simulink model "FLIGHT_Hexacopter_fail"  (R2024a)
settings: Solver=FixedStepDiscrete  StartTime=0.0  StopTime=inf  FixedStep=SampleTime  RelTol=1e-3  EnableMultiTasking=on
InitFcn:
  | Init_FLIGHT_Hexacopter
values from neighbouring files (symbols this model uses):
  Kdpr = 0.004    [Init_FLIGHT_Hexacopter_fromNCMS.m]
  Kdrr = 0.004    [Init_FLIGHT_Hexacopter_fromNCMS.m]
  Kdvz = 0.0254    [Init_FLIGHT_Hexacopter_fromNCMS.m]
  Kdyr = 0.0298    [Init_FLIGHT_Hexacopter_fromNCMS.m]
  Kipr = 0.0    (= 0)    [Init_FLIGHT_Hexacopter_fromNCMS.m]
  Kirr = 0.0    (= 0)    [Init_FLIGHT_Hexacopter_fromNCMS.m]
  Kivz = 0.6304    [Init_FLIGHT_Hexacopter_fromNCMS.m]
  Kiyr = 0.0    (= 0)    [Init_FLIGHT_Hexacopter_fromNCMS.m]
  Kpp = 3.3894    [Init_FLIGHT_Hexacopter_fromNCMS.m]
  Kppr = 0.1    [Init_FLIGHT_Hexacopter_fromNCMS.m]
  Kpr = 3.3894    [Init_FLIGHT_Hexacopter_fromNCMS.m]
  Kprr = 0.1    [Init_FLIGHT_Hexacopter_fromNCMS.m]
  Kpvz = 0.3191    [Init_FLIGHT_Hexacopter_fromNCMS.m]
  Kpyr = 0.3744    [Init_FLIGHT_Hexacopter_fromNCMS.m]
  MAX_CONTROL_ANGLE_PITCH = 30*pi/180    (= 0.523598775598)    [Init_FLIGHT_Hexacopter.m]    (also in Init_FLIGHT_Hexacopter_fromNCMS.m = 0.349065850399)
  MAX_CONTROL_ANGLE_RATE_PITCH = 360*pi/180    (= 6.28318530718)    [Init_FLIGHT_Hexacopter.m]    (also in Init_FLIGHT_Hexacopter_fromNCMS.m)
  MAX_CONTROL_ANGLE_RATE_ROLL = 360*pi/180    (= 6.28318530718)    [Init_FLIGHT_Hexacopter.m]    (also in Init_FLIGHT_Hexacopter_fromNCMS.m)
  MAX_CONTROL_ANGLE_RATE_Y = 120*pi/180    (= 2.09439510239)    [Init_FLIGHT_Hexacopter.m]    (also in Init_FLIGHT_Hexacopter_fromNCMS.m)
  MAX_CONTROL_ANGLE_ROLL = 30*pi/180    (= 0.523598775598)    [Init_FLIGHT_Hexacopter.m]    (also in Init_FLIGHT_Hexacopter_fromNCMS.m = 0.349065850399)
  MAX_CONTROL_VELOCITY_Z = 1    [Init_FLIGHT_Hexacopter.m]    (also in Init_FLIGHT_Hexacopter_fromNCMS.m)
  Npr = 50    [Init_FLIGHT_Hexacopter_fromNCMS.m]
  Nrr = 50    [Init_FLIGHT_Hexacopter_fromNCMS.m]
  Nvz = Npr    (= 50)    [Init_FLIGHT_Hexacopter_fromNCMS.m]
  Nyr = 50    [Init_FLIGHT_Hexacopter_fromNCMS.m]
  SampleTime = 1/250    (= 0.004)    [Init_FLIGHT_Hexacopter.m]    (also in Init_FLIGHT_Hexacopter_fromNCMS.m = 0.01)
  THR_HOVER = 0.6085    [Init_FLIGHT_Hexacopter_fromNCMS.m]
libraries: px4lib x7, slpidlib x6, px4Sensorslib x3, simulink x2, px4uORBlib x1
(part 1 of 2)
settings Model: ExtModeTrigDuration=10  Creator=user  LastModifiedBy=user
settings SolverCC: PositivePriorityOrder=on
settings OptimizationCC: DefaultUnderspecifiedDataType=single  EnhancedBackFolding=on  PassReuseOutputArgsAs=Individual arguments  ZeroExternalMemoryAtStartup=off  ZeroInternalMemoryAtStartup=off  MaxStackSize=64  OptimizeBlockOrder=speed  DifferentSizesBufferReuse=on  OptimizationCustomize=off  EfficientTunableParamExpr=on
settings DebuggingCC: ParameterTunabilityLossMsg=error  UnconnectedInputMsg=warning  UnconnectedOutputMsg=warning  UnconnectedLineMsg=warning
settings HardwareCC: ProdBitPerPointer=32  ProdBitPerSizeT=32  ProdBitPerPtrDiffT=32  ProdLargestAtomicInteger=Long  ProdLargestAtomicFloat=Double  ProdWordSize=32  ProdLongLongMode=on  ProdHWDeviceType=ARM Compatible->ARM Cortex
settings ModelReferenceCC: EnableRefExpFcnMdlSchedulingChecks=on
settings SFSimCC: MATLABDynamicMemAlloc=off  SimTargetLang=C++
settings RTWCC: Description=Embedded Coder  SystemTargetFile=ert.tlc  HardwareBoard=PX4 Cube Orange  TLCOptions="-aInlineSetEventsForThisBaseRateFcn=TLC_FALSE -aSuppressMultiTaskScheduler=TLC_FALSE  -aRateBasedStepFcn=0"  TemplateMakefile=ert_default_tmf  Toolchain=GNU Tools for PX4 Autopilots  TargetLang=C++  GPUComputeCapability=3.5  DLArmComputeVersion=19.05
settings CodeAppCC: ForceParamTrailComments=on  IgnoreCustomStorageClasses=off  OperatorAnnotations=on  SimulinkDataObjDesc=on  SFDataObjDesc=on  InsertBlockDesc=on
settings ERTTargetCC: MatFileLogging=on  ExtModeTransport=3  ExtModeStaticAlloc=on  ExtModeStaticAllocSize=1024  ExtModeMexFile=ext_xcp  ExtModeIntrfLevel=Level2 - Open

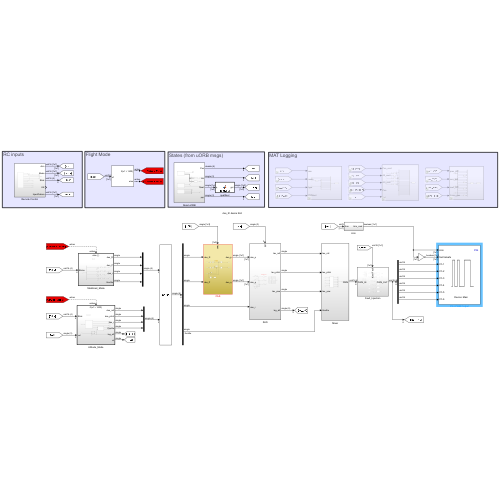
[thumbnail: Simulink's stored preview of the top-level diagram]
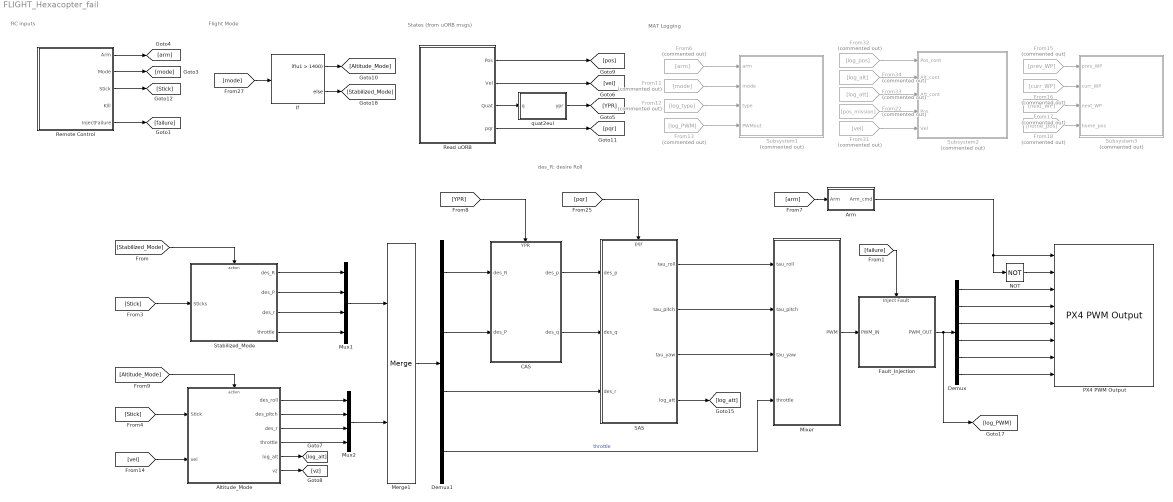
== system FLIGHT_Hexacopter_fail ==
  note: des_R: desire Roll
  note: MAT Logging
  note: States (from uORB msgs)
  note: RC inputs
  note: Flight Mode
  Altitude_Mode : Subsystem
  Arm : Subsystem
  CAS : Subsystem
      settings: PortSchema="{\"entries\":[{\"content\":{\"sides\":[{\"content\":{\"connectorIds\":[\"In1\",\"In2\"]},\"type\":\"ConnectorPlacement.EquallySpacedRectSide\",\"uuid\":\"cd8887f4-d1ed-4900-9f4b-1d4d1f8b3f25\"},{\"content\":{\"connectorIds\":[\"Out1\",\"Out2\"],\"side\":\"RIGHT\"},\"type\":\"ConnectorPlacement.EquallySpacedRectSide\",\"uuid\":\"04130072-6486-422d-805d-1cc854b52651\"},{\"content\":{\"connectorIds\":[\"In3\"],\"side\":\"TOP\"},\"type\":\"ConnectorPlacement.EquallySpacedRectSide\",\"uuid\":\"bd75db6e-c74e-4c5f-b850-7d60a52ba57c\"}]},\"type\":\"ConnectorPlacement.EquallySpacedConnector\",\"uuid\":\"0b75b304-9bf2-4ad4-968c-84bda26ed250\"}],\"packageUris\":[\"http://schema.mathworks.com/mf0/Connector/R2020b\"],\"version\":\"1.0\"}"
  Demux : Demux  Outputs=6
  Demux1 : Demux
  Fault_Injection : Subsystem
      settings: PortSchema="{\"entries\":[{\"content\":{\"sides\":[{\"content\":{\"connectorIds\":[\"In1\"]},\"type\":\"ConnectorPlacement.EquallySpacedRectSide\",\"uuid\":\"fab26c65-8d77-46b7-b375-2033d08e8306\"},{\"content\":{\"connectorIds\":[\"Out1\"],\"side\":\"RIGHT\"},\"type\":\"ConnectorPlacement.EquallySpacedRectSide\",\"uuid\":\"bc3f50bd-e170-4b75-8089-4f92da68e83e\"},{\"content\":{\"connectorIds\":[\"In2\"],\"side\":\"TOP\"},\"type\":\"ConnectorPlacement.EquallySpacedRectSide\",\"uuid\":\"873ada90-6f93-48ab-a701-a52d28357753\"}]},\"type\":\"ConnectorPlacement.EquallySpacedConnector\",\"uuid\":\"201be8b3-bff4-4924-8e0c-28e5fee33d1c\"}],\"packageUris\":[\"http://schema.mathworks.com/mf0/Connector/R2020b\"],\"version\":\"1.0\"}"
  From11 : From  Commented=on  GotoTag=mode
  From12 : From  Commented=on  GotoTag=log_type
  From13 : From  Commented=on  GotoTag=log_PWM
  From15 : From  Commented=on  GotoTag=prev_WP
  From16 : From  Commented=on  GotoTag=curr_WP
  From17 : From  Commented=on  GotoTag=next_WP
  From18 : From  Commented=on  GotoTag=home_pos
  From22 : From  Commented=on  GotoTag=pos_mission
  From31 : From  Commented=on  GotoTag=vel
  From32 : From  Commented=on  GotoTag=log_pos
  From33 : From  Commented=on  GotoTag=log_att
  From34 : From  Commented=on  GotoTag=log_alt
  From6 : From  Commented=on  GotoTag=arm
  If : If  IfExpression=u1 > 1400
  Merge1 : Merge
  Mixer : Subsystem
  Mux1 : Mux
  Mux2 : Mux
  NOT : Logic  Operator=NOT  IconShape=distinctive  AllPortsSameDT=off  OutDataTypeStr=boolean
  PX4 PWM Output : px4lib/PX4 PWM Output  pwmDevice=Main  pwmChannel1_=on  pwmChannel2_=on  pwmChannel3_=on  pwmChannel4_=on  pwmChannel5_=on  pwmChannel6_=on  pwmChannel7_=off  pwmChannel8_=off
  Read uORB : Subsystem
  Remote Control : Subsystem
  SAS : Subsystem
      settings: PortSchema="{\"entries\":[{\"content\":{\"sides\":[{\"content\":{\"connectorIds\":[\"In1\",\"In2\",\"In3\"]},\"type\":\"ConnectorPlacement.EquallySpacedRectSide\",\"uuid\":\"77bb8164-b871-4593-8031-335c6110c17c\"},{\"content\":{\"connectorIds\":[\"Out1\",\"Out2\",\"Out3\",\"Out4\"],\"side\":\"RIGHT\"},\"type\":\"ConnectorPlacement.EquallySpacedRectSide\",\"uuid\":\"f99d9e85-7cc9-4d0a-ad5d-789571e28028\"},{\"content\":{\"connectorIds\":[\"In4\"],\"side\":\"TOP\"},\"type\":\"ConnectorPlacement.EquallySpacedRectSide\",\"uuid\":\"174eb658-0f52-43c7-ba1a-1a337b4835ca\"}]},\"type\":\"ConnectorPlacement.EquallySpacedConnector\",\"uuid\":\"7932b1f4-42ae-4dcf-8815-0888db42261d\"}],\"packageUris\":[\"http://schema.mathworks.com/mf0/Connector/R2020b\"],\"version\":\"1.0\"}"
  Stabilized_Mode : Subsystem  TreatAsAtomicUnit=on
  Subsystem1 : Subsystem  Commented=on
  Subsystem2 : Subsystem  Commented=on
  Subsystem3 : Subsystem  Commented=on
  quat2eul : MATLAB Function  TreatAsAtomicUnit=on
  wires:
  Demux/1 -> PX4 PWM Output/3
  Demux/2 -> PX4 PWM Output/4
  Demux/3 -> PX4 PWM Output/5
  Demux/4 -> PX4 PWM Output/6
  NOT/1 -> PX4 PWM Output/2
  Read uORB/3(Quat) -> quat2eul/1(q)
  Arm/1(Arm_cmd) -> NOT/1, PX4 PWM Output/1
  Read uORB/2(Vel) -> [vel]
  Remote Control/3(Stick) -> [Stick]
  Remote Control/2(Mode) -> [mode]
  Remote Control/1(Arm) -> [arm]
  Read uORB/1(Pos) -> [pos]
  Merge1/1 -> Demux1/1
  [arm] -> Arm/1(Arm)
  quat2eul/1(ypr) -> [YPR]
  Read uORB/4(pqr) -> [pqr]
  SAS/4(log_att) -> [log_att]
  From6/1 -> Subsystem1/1(arm)
  From11/1 -> Subsystem1/2(mode)
  From12/1 -> Subsystem1/3(type)
  From13/1 -> Subsystem1/4(PWMout)
  [pqr] -> SAS/4(pqr)
  From31/1 -> Subsystem2/5(Vel)
  From22/1 -> Subsystem2/4(Pos)
  From33/1 -> Subsystem2/3(Att_cont)
  From34/1 -> Subsystem2/2(Alt_cont)
  From32/1 -> Subsystem2/1(Pos_cont)
  From18/1 -> Subsystem3/4(home_pos)
  From17/1 -> Subsystem3/3(next_WP)
  From16/1 -> Subsystem3/2(curr_WP)
  From15/1 -> Subsystem3/1(prev_WP)
  Demux/5 -> PX4 PWM Output/7
  Demux/6 -> PX4 PWM Output/8
  [mode] -> If/1
  Demux1/2 -> CAS/2(des_P)
  Demux1/1 -> CAS/1(des_R)
  [YPR] -> CAS/3(YPR)
  [Stabilized_Mode] -> Stabilized_Mode/Action
  [Stick] -> Stabilized_Mode/1(Sticks)
  Mux1/1 -> Merge1/1
  CAS/1(des_p) -> SAS/1(des_p)
  CAS/2(des_q) -> SAS/2(des_q)
  Demux1/3 -> SAS/3(des_r)
  Demux1/4 -> Mixer/4(throttle)  "throttle"
  [Stick] -> Altitude_Mode/1(Stick)
  [Altitude_Mode] -> Altitude_Mode/Action
  Altitude_Mode/1(des_roll) -> Mux2/1
  Altitude_Mode/2(des_pitch) -> Mux2/2
  Altitude_Mode/3(des_r) -> Mux2/3
  Altitude_Mode/4(throttle) -> Mux2/4
  Mux2/1 -> Merge1/2
  Altitude_Mode/5(log_alt) -> [log_alt]
  Altitude_Mode/6(vz) -> [vz]
  [vel] -> Altitude_Mode/2(vel)
  SAS/1(tau_roll) -> Mixer/1(tau_roll)
  SAS/2(tau_pitch) -> Mixer/2(tau_pitch)
  SAS/3(tau_yaw) -> Mixer/3(tau_yaw)
  Mixer/1(PWM) -> Fault_Injection/1(PWM_IN)
  Fault_Injection/1(PWM_OUT) -> [log_PWM], Demux/1
  Remote Control/5(InjectFailure) -> [failure]
  [failure] -> Fault_Injection/2(Inject Fault)
  If/1 -> [Altitude_Mode]
  If/2 -> [Stabilized_Mode]
  Stabilized_Mode/1(des_R) -> Mux1/1
  Stabilized_Mode/2(des_P) -> Mux1/2
  Stabilized_Mode/3(des_r) -> Mux1/3
  Stabilized_Mode/4(throttle) -> Mux1/4

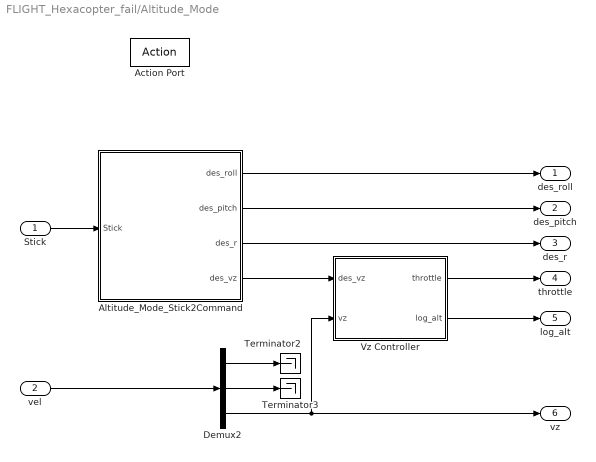
== system FLIGHT_Hexacopter_fail/Altitude_Mode ==
  Stick : Inport
  vel : Inport  Port=2
  Action Port : ActionPort  ActionPortLabel=if(u1 > 1400)
  Altitude_Mode_Stick2Command : Subsystem
  Demux2 : Demux  Outputs=3
  Terminator2 : Terminator
  Terminator3 : Terminator
  Vz Controller : Subsystem
  des_roll : Outport
  des_pitch : Outport  Port=2
  des_r : Outport  Port=3
  throttle : Outport  Port=4
  log_alt : Outport  Port=5
  vz : Outport  Port=6
  wires:
  Stick/1 -> Altitude_Mode_Stick2Command/1(Stick)
  Vz Controller/1(throttle) -> throttle/1
  Demux2/3 -> vz/1, Vz Controller/2(vz)
  Altitude_Mode_Stick2Command/1(des_roll) -> des_roll/1
  vel/1 -> Demux2/1
  Altitude_Mode_Stick2Command/3(des_r) -> des_r/1
  Demux2/1 -> Terminator2/1
  Vz Controller/2(log_alt) -> log_alt/1
  Demux2/2 -> Terminator3/1
  Altitude_Mode_Stick2Command/2(des_pitch) -> des_pitch/1
  Altitude_Mode_Stick2Command/4(des_vz) -> Vz Controller/1(des_vz)

== system FLIGHT_Hexacopter_fail/Arm ==
  Arm : Inport
  Compare To Constant3 : simulink/Logic and Bit Operations/Compare To Constant  relop=>=  const=uint16(1800)  OutDataTypeStr=boolean
  Arm_cmd : Outport  VectorParamsAs1DForOutWhenUnconnected=off
  wires:
  Arm/1 -> Compare To Constant3/1
  Compare To Constant3/1 -> Arm_cmd/1

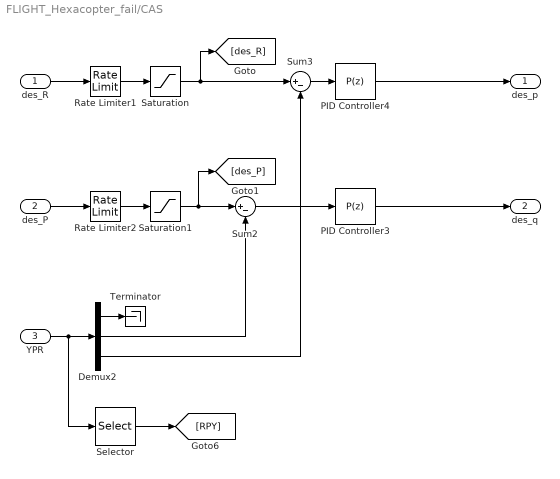
== system FLIGHT_Hexacopter_fail/CAS ==
  des_R : Inport
  des_P : Inport  Port=2
  YPR : Inport  Port=3
  Demux2 : Demux  Outputs=3
  PID Controller3 : slpidlib/PID Controller  Controller=P  Form=Parallel  TimeDomain=Discrete-time  UseExternalTs=off  SampleTime=SampleTime  IntegratorMethod=Forward Euler  FilterMethod=Forward Euler  ControllerParametersSource=internal  P=Kpp  I=1  UseKiTs=off  D=0  UseExternalDerivativeSource=off  N=100  UseFilter=on  TunerSelectOption=Transfer Function Based (PID Tuner App)  InitialConditionSource=internal  InitialConditionForIntegrator=0  InitialConditionForFilter=0  DifferentiatorICPrevScaledInput=0  ExternalReset=none  TrackingMode=off  Kt=1  LimitOutput=on  SatLimitsSource=internal  UpperSaturationLimit=MAX_CONTROL_ANGLE_RATE_PITCH  LowerSaturationLimit=-MAX_CONTROL_ANGLE_RATE_PITCH  LinearizeAsGain=on  AntiWindupMode=none  Kb=1  LimitIntegrator=off  UpperIntegratorSaturationLimit=inf  LowerIntegratorSaturationLimit=-inf  POutMin=[]  POutMax=[]  IOutMin=[]  IOutMax=[]  DOutMin=[]  DOutMax=[]  NOutMin=[]  NOutMax=[]  SumOutMin=[]  SumOutMax=[]  SaturationOutMin=[]  SaturationOutMax=[]  PParamMin=[]  PParamMax=[]  IParamMin=[]  IParamMax=[]  DParamMin=[]  DParamMax=[]  NParamMin=[]  NParamMax=[]  KbParamMin=[]  KbParamMax=[]  KtParamMin=[]  KtParamMax=[]  KbOutMin=[]  KbOutMax=[]  KtOutMin=[]  KtOutMax=[]  IntegratorOutMin=[]  IntegratorOutMax=[]  FilterOutMin=[]  FilterOutMax=[]  SumI1OutMin=[]  SumI1OutMax=[]  SumI2OutMin=[]  SumI2OutMax=[]  SumI3OutMin=[]  SumI3OutMax=[]  SumI4OutMin=[]  SumI4OutMax=[]  SumDOutMin=[]  SumDOutMax=[]  DifferentiatorOutMin=[]  DifferentiatorOutMax=[]  FilterDiffOutCoefMin=[]  FilterDiffOutCoefMax=[]  ReciprocalOutMin=[]  ReciprocalOutMax=[]  SumDenOutMin=[]  SumDenOutMax=[]  SumNumOutMin=[]  SumNumOutMax=[]  DivideOutMin=[]  DivideOutMax=[]  UdiffTsProdOutMin=[]  UdiffTsProdOutMax=[]  NTsProdOutMin=[]  NTsProdOutMax=[]  UintegralTsProdOutMin=[]  UintegralTsProdOutMax=[]  UngainTsProdOutMin=[]  UngainTsProdOutMax=[]  ClampingZeroOutDataTypeStr=Inherit: Inherit via back propagation  ClampingZeroOutMin=[]  ClampingZeroOutMax=[]  FilterDenConstantOutDataTypeStr=Inherit: Inherit via back propagation  FilterDenConstantOutMin=[]  FilterDenConstantOutMax=[]  PCopyOutDataTypeStr=Inherit: Inherit via back propagation  PCopyOutMin=[]  PCopyOutMax=[]  NCopyOutDataTypeStr=Inherit: Inherit via back propagation  NCopyOutMin=[]  NCopyOutMax=[]  IntegratorContinuousStateAttributes=''  IntegratorStateMustResolveToSignalObject=off  IntegratorRTWStateStorageClass=Auto  FilterContinuousStateAttributes=''  FilterStateMustResolveToSignalObject=off  FilterRTWStateStorageClass=Auto  ParallelPVariant=InternalParameters  IdealPVariant=Disabled  IVariant=Disabled  DVariant=Disabled  IntegratorVariant=Disabled  SatVariant=Enabled  AWVariant=Disabled  PCopyVariant=Disabled  TRVariant=Disabled  FdbkBlocksVariant=Forward  IdealPFdbkVariant=Disabled  SatFdbkVariant=Disabled  DerivativeFilterVariant=Disabled  NVariant=Disabled  NCopyVariant=Disabled_SignalSpec  FilterICVariant=Disabled  IntegratorICVariant=Disabled  ExternalResetVariant=Disabled  TRSumVariant=Passthrough  SumFdbkVariant=Disabled  SumVariant=Passthrough_P  TsampFilterVariant=InternalTs  TsampNgainVariant=Passthrough  TsampIntegralVariant=Disabled_SignalSpec  ExternalSaturationOutDataTypeStr=Inherit: Same as second input  DerivativeSourceVariant=Disabled
  PID Controller4 : slpidlib/PID Controller  Controller=P  Form=Parallel  TimeDomain=Discrete-time  UseExternalTs=off  SampleTime=SampleTime  IntegratorMethod=Forward Euler  FilterMethod=Forward Euler  ControllerParametersSource=internal  P=Kpr  I=1  UseKiTs=off  D=0  UseExternalDerivativeSource=off  N=100  UseFilter=on  TunerSelectOption=Transfer Function Based (PID Tuner App)  InitialConditionSource=internal  InitialConditionForIntegrator=0  InitialConditionForFilter=0  DifferentiatorICPrevScaledInput=0  ExternalReset=none  TrackingMode=off  Kt=1  LimitOutput=on  SatLimitsSource=internal  UpperSaturationLimit=MAX_CONTROL_ANGLE_RATE_ROLL  LowerSaturationLimit=-MAX_CONTROL_ANGLE_RATE_ROLL  LinearizeAsGain=on  AntiWindupMode=none  Kb=1  LimitIntegrator=off  UpperIntegratorSaturationLimit=inf  LowerIntegratorSaturationLimit=-inf  POutMin=[]  POutMax=[]  IOutMin=[]  IOutMax=[]  DOutMin=[]  DOutMax=[]  NOutMin=[]  NOutMax=[]  SumOutMin=[]  SumOutMax=[]  SaturationOutMin=[]  SaturationOutMax=[]  PParamMin=[]  PParamMax=[]  IParamMin=[]  IParamMax=[]  DParamMin=[]  DParamMax=[]  NParamMin=[]  NParamMax=[]  KbParamMin=[]  KbParamMax=[]  KtParamMin=[]  KtParamMax=[]  KbOutMin=[]  KbOutMax=[]  KtOutMin=[]  KtOutMax=[]  IntegratorOutMin=[]  IntegratorOutMax=[]  FilterOutMin=[]  FilterOutMax=[]  SumI1OutMin=[]  SumI1OutMax=[]  SumI2OutMin=[]  SumI2OutMax=[]  SumI3OutMin=[]  SumI3OutMax=[]  SumI4OutMin=[]  SumI4OutMax=[]  SumDOutMin=[]  SumDOutMax=[]  DifferentiatorOutMin=[]  DifferentiatorOutMax=[]  FilterDiffOutCoefMin=[]  FilterDiffOutCoefMax=[]  ReciprocalOutMin=[]  ReciprocalOutMax=[]  SumDenOutMin=[]  SumDenOutMax=[]  SumNumOutMin=[]  SumNumOutMax=[]  DivideOutMin=[]  DivideOutMax=[]  UdiffTsProdOutMin=[]  UdiffTsProdOutMax=[]  NTsProdOutMin=[]  NTsProdOutMax=[]  UintegralTsProdOutMin=[]  UintegralTsProdOutMax=[]  UngainTsProdOutMin=[]  UngainTsProdOutMax=[]  ClampingZeroOutDataTypeStr=Inherit: Inherit via back propagation  ClampingZeroOutMin=[]  ClampingZeroOutMax=[]  FilterDenConstantOutDataTypeStr=Inherit: Inherit via back propagation  FilterDenConstantOutMin=[]  FilterDenConstantOutMax=[]  PCopyOutDataTypeStr=Inherit: Inherit via back propagation  PCopyOutMin=[]  PCopyOutMax=[]  NCopyOutDataTypeStr=Inherit: Inherit via back propagation  NCopyOutMin=[]  NCopyOutMax=[]  IntegratorContinuousStateAttributes=''  IntegratorStateMustResolveToSignalObject=off  IntegratorRTWStateStorageClass=Auto  FilterContinuousStateAttributes=''  FilterStateMustResolveToSignalObject=off  FilterRTWStateStorageClass=Auto  ParallelPVariant=InternalParameters  IdealPVariant=Disabled  IVariant=Disabled  DVariant=Disabled  IntegratorVariant=Disabled  SatVariant=Enabled  AWVariant=Disabled  PCopyVariant=Disabled  TRVariant=Disabled  FdbkBlocksVariant=Forward  IdealPFdbkVariant=Disabled  SatFdbkVariant=Disabled  DerivativeFilterVariant=Disabled  NVariant=Disabled  NCopyVariant=Disabled_SignalSpec  FilterICVariant=Disabled  IntegratorICVariant=Disabled  ExternalResetVariant=Disabled  TRSumVariant=Passthrough  SumFdbkVariant=Disabled  SumVariant=Passthrough_P  TsampFilterVariant=InternalTs  TsampNgainVariant=Passthrough  TsampIntegralVariant=Disabled_SignalSpec  ExternalSaturationOutDataTypeStr=Inherit: Same as second input  DerivativeSourceVariant=Disabled
  Rate Limiter1 : RateLimiter  RisingSlewLimit=40*pi/180  FallingSlewLimit=-40*pi/180  SampleTimeMode=inherited
  Rate Limiter2 : RateLimiter  RisingSlewLimit=40*pi/180  FallingSlewLimit=-40*pi/180  SampleTimeMode=inherited
  Saturation : Saturate  UpperLimit=MAX_CONTROL_ANGLE_ROLL  LowerLimit=-MAX_CONTROL_ANGLE_ROLL
  Saturation1 : Saturate  UpperLimit=MAX_CONTROL_ANGLE_PITCH  LowerLimit=-MAX_CONTROL_ANGLE_PITCH
  Selector : Selector  InputPortWidth=3  IndexOptions=Index vector (dialog)  Indices=[3 2 1]  OutputSizes=1
  Sum2 : Sum  Inputs=|+-
  Sum3 : Sum  Inputs=|+-
  Terminator : Terminator
  des_p : Outport
  des_q : Outport  Port=2
  wires:
  des_R/1 -> Rate Limiter1/1
  Saturation/1 -> [des_R], Sum3/1
  Sum3/1 -> PID Controller4/1
  Sum2/1 -> PID Controller3/1
  Saturation1/1 -> [des_P], Sum2/1
  Demux2/3 -> Sum3/2
  Demux2/2 -> Sum2/2
  YPR/1 -> Selector/1, Demux2/1
  Selector/1 -> [RPY]
  Rate Limiter1/1 -> Saturation/1
  Demux2/1 -> Terminator/1
  des_P/1 -> Rate Limiter2/1
  Rate Limiter2/1 -> Saturation1/1
  PID Controller4/1 -> des_p/1
  PID Controller3/1 -> des_q/1

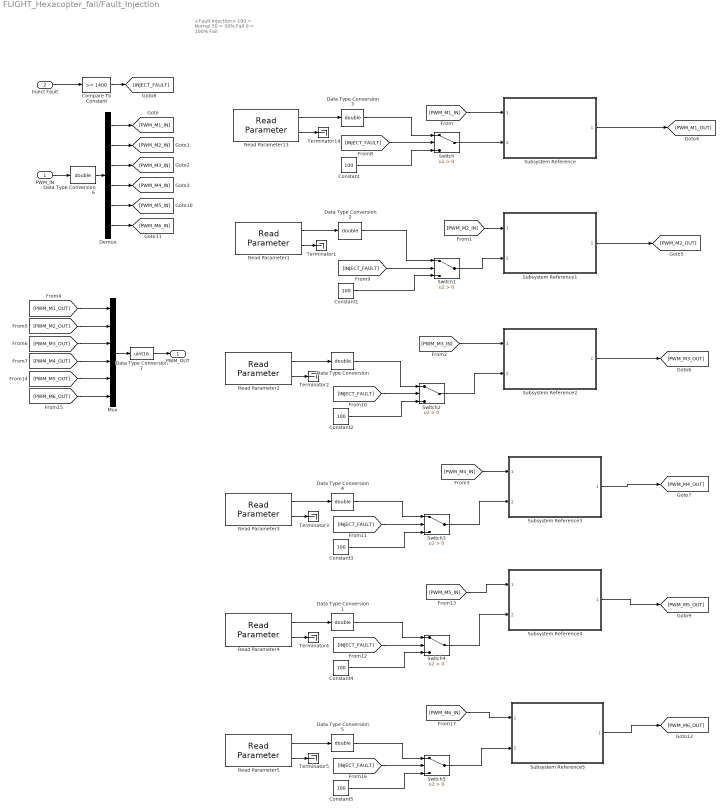
== system FLIGHT_Hexacopter_fail/Fault_Injection ==
  note: <Fault Injection>
      | 100 = Nornal
      | 50 = 50% Fail
      | 0 = 100% Fail
  PWM_IN : Inport
  Inject Fault : Inport  Port=2
  Compare To Constant : simulink/Logic and Bit Operations/Compare To Constant  relop=>=  const=1400  OutDataTypeStr=boolean
  Constant{,1..5} (6 alike) : Constant  Value=100
  Data Type Conversion{,1..6} (7 alike) : DataTypeConversion  OutDataTypeStr=double  SaturateOnIntegerOverflow=off  RndMeth=Floor
  Data Type Conversion7 : DataTypeConversion  OutDataTypeStr=uint16  SaturateOnIntegerOverflow=off  RndMeth=Floor
  Demux : Demux  Outputs=6
  Mux : Mux  Inputs=6
  Read Parameter1 : px4lib/Read Parameter  ParameterName=FDD_M2_STATUS  DataType=INT32  SampleTime=-1
  Read Parameter13 : px4lib/Read Parameter  ParameterName=FDD_M1_STATUS  DataType=INT32  SampleTime=-1
  Read Parameter2 : px4lib/Read Parameter  ParameterName=FDD_M3_STATUS  DataType=INT32  SampleTime=-1
  Read Parameter3 : px4lib/Read Parameter  ParameterName=FDD_M4_STATUS  DataType=INT32  SampleTime=-1
  Read Parameter4 : px4lib/Read Parameter  ParameterName=FDD_M5_STATUS  DataType=INT32  SampleTime=-1
  Read Parameter5 : px4lib/Read Parameter  ParameterName=FDD_M6_STATUS  DataType=INT32  SampleTime=-1
  Subsystem Reference{,1..5} (6 alike) : Subsystem  ReferencedSubsystem=calculate_fault_injected_pwm
  Switch{,1..5} (6 alike) : Switch  Criteria=u2 > Threshold  SaturateOnIntegerOverflow=off  InputSameDT=off
  Terminator{1..5,14} (6 alike) : Terminator
  PWM_OUT : Outport
  wires:
  Read Parameter13/2 -> Terminator14/1
  Read Parameter1/2 -> Terminator1/1
  Read Parameter2/2 -> Terminator2/1
  Read Parameter2/1 -> Data Type Conversion/1
  Read Parameter3/2 -> Terminator3/1
  Read Parameter3/1 -> Data Type Conversion4/1
  Read Parameter13/1 -> Data Type Conversion3/1
  Read Parameter1/1 -> Data Type Conversion2/1
  Demux/1 -> [PWM_M1_IN]
  Demux/2 -> [PWM_M2_IN]
  Demux/3 -> [PWM_M3_IN]
  Demux/4 -> [PWM_M4_IN]
  Mux/1 -> Data Type Conversion7/1
  [PWM_M1_OUT] -> Mux/1
  [PWM_M2_OUT] -> Mux/2
  [PWM_M3_OUT] -> Mux/3
  [PWM_M4_OUT] -> Mux/4
  Inject Fault/1 -> Compare To Constant/1
  Compare To Constant/1 -> [INJECT_FAULT]
  Data Type Conversion3/1 -> Switch/1
  [INJECT_FAULT] -> Switch/2
  Constant/1 -> Switch/3
  Constant1/1 -> Switch1/3
  [INJECT_FAULT] -> Switch1/2
  Constant2/1 -> Switch2/3
  [INJECT_FAULT] -> Switch2/2
  Data Type Conversion/1 -> Switch2/1
  Constant3/1 -> Switch3/3
  [INJECT_FAULT] -> Switch3/2
  Data Type Conversion4/1 -> Switch3/1
  Read Parameter4/1 -> Data Type Conversion1/1
  Data Type Conversion1/1 -> Switch4/1
  Constant4/1 -> Switch4/3
  Read Parameter4/2 -> Terminator4/1
  [INJECT_FAULT] -> Switch4/2
  Demux/5 -> [PWM_M5_IN]
  Demux/6 -> [PWM_M6_IN]
  [PWM_M5_OUT] -> Mux/5
  [PWM_M6_OUT] -> Mux/6
  Data Type Conversion5/1 -> Switch5/1
  Read Parameter5/2 -> Terminator5/1
  [INJECT_FAULT] -> Switch5/2
  Read Parameter5/1 -> Data Type Conversion5/1
  Constant5/1 -> Switch5/3
  Data Type Conversion2/1 -> Switch1/1
  [PWM_M1_IN] -> Subsystem Reference/1
  Switch/1 -> Subsystem Reference/2
  [PWM_M2_IN] -> Subsystem Reference1/1
  Switch1/1 -> Subsystem Reference1/2
  [PWM_M3_IN] -> Subsystem Reference2/1
  Switch2/1 -> Subsystem Reference2/2
  Switch3/1 -> Subsystem Reference3/2
  [PWM_M4_IN] -> Subsystem Reference3/1
  [PWM_M5_IN] -> Subsystem Reference4/1
  Switch4/1 -> Subsystem Reference4/2
  [PWM_M6_IN] -> Subsystem Reference5/1
  Switch5/1 -> Subsystem Reference5/2
  Subsystem Reference/1 -> [PWM_M1_OUT]
  Subsystem Reference1/1 -> [PWM_M2_OUT]
  Subsystem Reference2/1 -> [PWM_M3_OUT]
  Subsystem Reference3/1 -> [PWM_M4_OUT]
  Subsystem Reference4/1 -> [PWM_M5_OUT]
  Subsystem Reference5/1 -> [PWM_M6_OUT]
  Data Type Conversion6/1 -> Demux/1
  PWM_IN/1 -> Data Type Conversion6/1
  Data Type Conversion7/1 -> PWM_OUT/1

== system FLIGHT_Hexacopter_fail/Mixer ==
  tau_roll : Inport
  tau_pitch : Inport  Port=2
  tau_yaw : Inport  Port=3
  throttle : Inport  Port=4
  Mux : Mux  Inputs=6
  Output_Limits1 : Saturate  UpperLimit=2000  LowerLimit=1000  OutDataTypeStr=uint16
  pwm_out2 : MATLAB Function  SystemSampleTime=0.004
  PWM : Outport
  wires:
  tau_yaw/1 -> pwm_out2/3(Yaw)
  throttle/1 -> pwm_out2/4(Thrust)
  tau_roll/1 -> pwm_out2/1(Roll)
  pwm_out2/5(M5) -> Mux/5
  pwm_out2/6(M6) -> Mux/6
  tau_pitch/1 -> pwm_out2/2(Pitch)
  pwm_out2/4(M4) -> Mux/4
  pwm_out2/2(M2) -> Mux/2
  pwm_out2/3(M3) -> Mux/3
  pwm_out2/1(M1) -> Mux/1
  Output_Limits1/1 -> PWM/1
  Mux/1 -> Output_Limits1/1

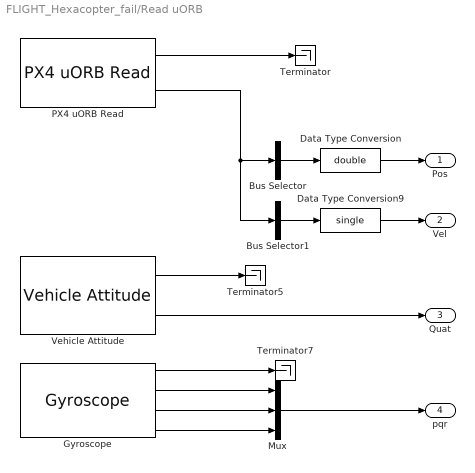
== system FLIGHT_Hexacopter_fail/Read uORB ==
  Bus Selector : BusSelector  OutputSignals=x,y,z,heading  OutputAsBus=on
  Bus Selector1 : BusSelector  OutputSignals=vx,vy,vz  OutputAsBus=on
  Data Type Conversion : DataTypeConversion  OutDataTypeStr=double  SaturateOnIntegerOverflow=off  RndMeth=Floor
  Data Type Conversion9 : DataTypeConversion  OutDataTypeStr=single  SaturateOnIntegerOverflow=off  RndMeth=Floor
  Gyroscope : px4Sensorslib/Gyroscope  uorbTimeStamp=off  BlockingMode=off  BlockTimeout=1e-3  sampleTime=SampleTime
  Mux : Mux  Inputs=3
  PX4 uORB Read : px4uORBlib/PX4 uORB Read  uORBTopic=VehicleLocalPosition  selectInstance=vehicle_local_position  SampleTime=SampleTime  BlockingMode=off  BlockTimeout=1e-3
  Terminator : Terminator
  Terminator5 : Terminator
  Terminator7 : Terminator
  Vehicle Attitude : px4Sensorslib/Vehicle Attitude  rollRate=off  pitchRate=off  yawRate=off  quaternion=on  uorbTimeStamp=off  BlockingMode=off  BlockTimeout=0.001  sampleTime=SampleTime
  Pos : Outport
  Vel : Outport  Port=2
  Quat : Outport  Port=3
  pqr : Outport  Port=4
  wires:
  Vehicle Attitude/1 -> Terminator5/1
  Gyroscope/4 -> Mux/3
  Gyroscope/3 -> Mux/2
  Gyroscope/2 -> Mux/1
  Gyroscope/1 -> Terminator7/1
  PX4 uORB Read/1 -> Terminator/1
  PX4 uORB Read/2 -> Bus Selector1/1, Bus Selector/1
  Mux/1 -> pqr/1
  Vehicle Attitude/2 -> Quat/1
  Bus Selector1/1 -> Data Type Conversion9/1
  Bus Selector/1 -> Data Type Conversion/1
  Data Type Conversion/1 -> Pos/1
  Data Type Conversion9/1 -> Vel/1

== system FLIGHT_Hexacopter_fail/Remote Control ==
  Mux3 : Mux
  Radio Control Transmitter : px4Sensorslib/Radio Control Transmitter  channel1=on  channel2=on  channel3=on  channel4=on  channel5=on  channel6=on  channel7=on  channel8=on  channel_count=off  rssi=off  rc_input_source=off  timestamp_last_signal=off  time_stamp=off  sampleTime=SampleTime  BlockingMode=off  BlockTimeout=5
  Terminator1 : Terminator
  Arm : Outport
  Mode : Outport  Port=2
  Stick : Outport  Port=3
  Kill : Outport  Port=4
  InjectFailure : Outport  Port=5
  wires:
  Radio Control Transmitter/6 -> Arm/1  "arm_signal"
  Mux3/1 -> Stick/1
  Radio Control Transmitter/1 -> Terminator1/1
  Radio Control Transmitter/7 -> Mode/1  "mode_signal"
  Radio Control Transmitter/5 -> Mux3/3  "des_Y"
  Radio Control Transmitter/4 -> Mux3/4  "throttle, des_vz"
  Radio Control Transmitter/8 -> Kill/1
  Radio Control Transmitter/9 -> InjectFailure/1
  Radio Control Transmitter/2 -> Mux3/1  "des_R"
  Radio Control Transmitter/3 -> Mux3/2  "des_P"

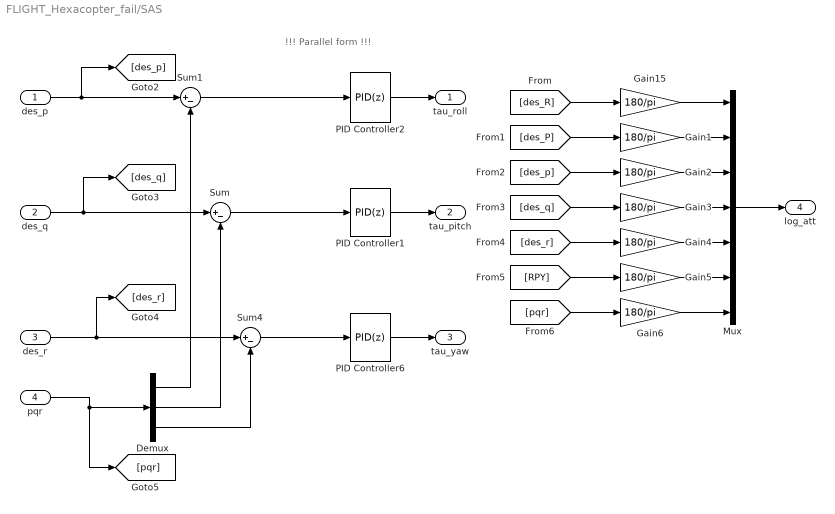
== system FLIGHT_Hexacopter_fail/SAS ==
  note: !!! Parallel form !!!
  des_p : Inport
  des_q : Inport  Port=2
  des_r : Inport  Port=3
  pqr : Inport  Port=4
  Demux : Demux  Outputs=3
  Gain{1..6,15} (7 alike) : Gain  Gain=180/pi
  Mux : Mux  Inputs=7
  PID Controller1 : slpidlib/PID Controller  Controller=PID  Form=Parallel  TimeDomain=Discrete-time  UseExternalTs=off  SampleTime=SampleTime  IntegratorMethod=Forward Euler  FilterMethod=Forward Euler  ControllerParametersSource=internal  P=Kppr  I=Kipr  UseKiTs=on  D=Kdpr  UseExternalDerivativeSource=off  N=Npr  UseFilter=on  TunerSelectOption=Transfer Function Based (PID Tuner App)  InitialConditionSource=internal  InitialConditionForIntegrator=0  InitialConditionForFilter=0  DifferentiatorICPrevScaledInput=0  ExternalReset=none  TrackingMode=off  Kt=1  LimitOutput=on  SatLimitsSource=internal  UpperSaturationLimit=0.2  LowerSaturationLimit=-0.2  LinearizeAsGain=on  AntiWindupMode=clamping  Kb=1  LimitIntegrator=off  UpperIntegratorSaturationLimit=inf  LowerIntegratorSaturationLimit=-inf  POutMin=[]  POutMax=[]  IOutMin=[]  IOutMax=[]  DOutMin=[]  DOutMax=[]  NOutMin=[]  NOutMax=[]  SumOutMin=[]  SumOutMax=[]  SaturationOutDataTypeStr=single  SaturationOutMin=[]  SaturationOutMax=[]  PParamMin=[]  PParamMax=[]  IParamMin=[]  IParamMax=[]  DParamMin=[]  DParamMax=[]  NParamMin=[]  NParamMax=[]  KbParamMin=[]  KbParamMax=[]  KtParamMin=[]  KtParamMax=[]  KbOutMin=[]  KbOutMax=[]  KtOutMin=[]  KtOutMax=[]  IntegratorOutMin=[]  IntegratorOutMax=[]  FilterOutMin=[]  FilterOutMax=[]  SumI1OutMin=[]  SumI1OutMax=[]  SumI2OutMin=[]  SumI2OutMax=[]  SumI3OutMin=[]  SumI3OutMax=[]  SumI4OutMin=[]  SumI4OutMax=[]  SumDOutMin=[]  SumDOutMax=[]  DifferentiatorOutMin=[]  DifferentiatorOutMax=[]  FilterDiffOutCoefMin=[]  FilterDiffOutCoefMax=[]  ReciprocalOutMin=[]  ReciprocalOutMax=[]  SumDenOutMin=[]  SumDenOutMax=[]  SumNumOutMin=[]  SumNumOutMax=[]  DivideOutMin=[]  DivideOutMax=[]  UdiffTsProdOutMin=[]  UdiffTsProdOutMax=[]  NTsProdOutMin=[]  NTsProdOutMax=[]  UintegralTsProdOutMin=[]  UintegralTsProdOutMax=[]  UngainTsProdOutMin=[]  UngainTsProdOutMax=[]  ClampingZeroOutDataTypeStr=Inherit: Inherit via back propagation  ClampingZeroOutMin=[]  ClampingZeroOutMax=[]  FilterDenConstantOutDataTypeStr=Inherit: Inherit via back propagation  FilterDenConstantOutMin=[]  FilterDenConstantOutMax=[]  PCopyOutDataTypeStr=Inherit: Inherit via back propagation  PCopyOutMin=[]  PCopyOutMax=[]  NCopyOutDataTypeStr=Inherit: Inherit via back propagation  NCopyOutMin=[]  NCopyOutMax=[]  IntegratorContinuousStateAttributes=''  IntegratorStateMustResolveToSignalObject=off  IntegratorRTWStateStorageClass=Auto  FilterContinuousStateAttributes=''  FilterStateMustResolveToSignalObject=off  FilterRTWStateStorageClass=Auto  ParallelPVariant=InternalParameters  IdealPVariant=Disabled  IVariant=InternalParameters  DVariant=InternalParameters  IntegratorVariant=Discrete  SatVariant=Enabled  AWVariant=DiscClampingParallel  PCopyVariant=Disabled  TRVariant=Disabled  FdbkBlocksVariant=Forward  IdealPFdbkVariant=Disabled  SatFdbkVariant=Disabled  DerivativeFilterVariant=ForwardEulerFilter  NVariant=InternalParameters  NCopyVariant=Disabled  FilterICVariant=InternalICsFilter  IntegratorICVariant=InternalICs  ExternalResetVariant=Disabled  TRSumVariant=Passthrough  SumFdbkVariant=Disabled  SumVariant=Sum_PID  TsampFilterVariant=InternalTs  TsampNgainVariant=Passthrough  TsampIntegralVariant=Disabled_SignalSpec  ExternalSaturationOutDataTypeStr=Inherit: Same as second input  DerivativeSourceVariant=ErrorSignal
  PID Controller2 : slpidlib/PID Controller  Controller=PID  Form=Parallel  TimeDomain=Discrete-time  UseExternalTs=off  SampleTime=SampleTime  IntegratorMethod=Forward Euler  FilterMethod=Forward Euler  ControllerParametersSource=internal  P=Kprr  I=Kirr  UseKiTs=on  D=Kdrr  UseExternalDerivativeSource=off  N=Nrr  UseFilter=on  TunerSelectOption=Transfer Function Based (PID Tuner App)  InitialConditionSource=internal  InitialConditionForIntegrator=0  InitialConditionForFilter=0  DifferentiatorICPrevScaledInput=0  ExternalReset=none  TrackingMode=off  Kt=1  LimitOutput=on  SatLimitsSource=internal  UpperSaturationLimit=0.2  LowerSaturationLimit=-0.2  LinearizeAsGain=on  AntiWindupMode=clamping  Kb=1  LimitIntegrator=off  UpperIntegratorSaturationLimit=inf  LowerIntegratorSaturationLimit=-inf  POutMin=[]  POutMax=[]  IOutMin=[]  IOutMax=[]  DOutMin=[]  DOutMax=[]  NOutMin=[]  NOutMax=[]  SumOutMin=[]  SumOutMax=[]  SaturationOutDataTypeStr=single  SaturationOutMin=[]  SaturationOutMax=[]  PParamMin=[]  PParamMax=[]  IParamMin=[]  IParamMax=[]  DParamMin=[]  DParamMax=[]  NParamMin=[]  NParamMax=[]  KbParamMin=[]  KbParamMax=[]  KtParamMin=[]  KtParamMax=[]  KbOutMin=[]  KbOutMax=[]  KtOutMin=[]  KtOutMax=[]  IntegratorOutMin=[]  IntegratorOutMax=[]  FilterOutMin=[]  FilterOutMax=[]  SumI1OutMin=[]  SumI1OutMax=[]  SumI2OutMin=[]  SumI2OutMax=[]  SumI3OutMin=[]  SumI3OutMax=[]  SumI4OutMin=[]  SumI4OutMax=[]  SumDOutMin=[]  SumDOutMax=[]  DifferentiatorOutMin=[]  DifferentiatorOutMax=[]  FilterDiffOutCoefMin=[]  FilterDiffOutCoefMax=[]  ReciprocalOutMin=[]  ReciprocalOutMax=[]  SumDenOutMin=[]  SumDenOutMax=[]  SumNumOutMin=[]  SumNumOutMax=[]  DivideOutMin=[]  DivideOutMax=[]  UdiffTsProdOutMin=[]  UdiffTsProdOutMax=[]  NTsProdOutMin=[]  NTsProdOutMax=[]  UintegralTsProdOutMin=[]  UintegralTsProdOutMax=[]  UngainTsProdOutMin=[]  UngainTsProdOutMax=[]  ClampingZeroOutDataTypeStr=Inherit: Inherit via back propagation  ClampingZeroOutMin=[]  ClampingZeroOutMax=[]  FilterDenConstantOutDataTypeStr=Inherit: Inherit via back propagation  FilterDenConstantOutMin=[]  FilterDenConstantOutMax=[]  PCopyOutDataTypeStr=Inherit: Inherit via back propagation  PCopyOutMin=[]  PCopyOutMax=[]  NCopyOutDataTypeStr=Inherit: Inherit via back propagation  NCopyOutMin=[]  NCopyOutMax=[]  IntegratorContinuousStateAttributes=''  IntegratorStateMustResolveToSignalObject=off  IntegratorRTWStateStorageClass=Auto  FilterContinuousStateAttributes=''  FilterStateMustResolveToSignalObject=off  FilterRTWStateStorageClass=Auto  ParallelPVariant=InternalParameters  IdealPVariant=Disabled  IVariant=InternalParameters  DVariant=InternalParameters  IntegratorVariant=Discrete  SatVariant=Enabled  AWVariant=DiscClampingParallel  PCopyVariant=Disabled  TRVariant=Disabled  FdbkBlocksVariant=Forward  IdealPFdbkVariant=Disabled  SatFdbkVariant=Disabled  DerivativeFilterVariant=ForwardEulerFilter  NVariant=InternalParameters  NCopyVariant=Disabled  FilterICVariant=InternalICsFilter  IntegratorICVariant=InternalICs  ExternalResetVariant=Disabled  TRSumVariant=Passthrough  SumFdbkVariant=Disabled  SumVariant=Sum_PID  TsampFilterVariant=InternalTs  TsampNgainVariant=Passthrough  TsampIntegralVariant=Disabled_SignalSpec  ExternalSaturationOutDataTypeStr=Inherit: Same as second input  DerivativeSourceVariant=ErrorSignal
  PID Controller6 : slpidlib/PID Controller  Controller=PID  Form=Parallel  TimeDomain=Discrete-time  UseExternalTs=off  SampleTime=SampleTime  IntegratorMethod=Forward Euler  FilterMethod=Forward Euler  ControllerParametersSource=internal  P=Kpyr  I=Kiyr  UseKiTs=on  D=Kdyr  UseExternalDerivativeSource=off  N=Nyr  UseFilter=on  TunerSelectOption=Transfer Function Based (PID Tuner App)  InitialConditionSource=internal  InitialConditionForIntegrator=0  InitialConditionForFilter=0  DifferentiatorICPrevScaledInput=0  ExternalReset=none  TrackingMode=off  Kt=1  LimitOutput=on  SatLimitsSource=internal  UpperSaturationLimit=0.4  LowerSaturationLimit=-0.4  LinearizeAsGain=on  AntiWindupMode=clamping  Kb=1  LimitIntegrator=off  UpperIntegratorSaturationLimit=inf  LowerIntegratorSaturationLimit=-inf  PGainOutDataTypeStr=single  PProdOutDataTypeStr=single  POutMin=[]  POutMax=[]  IGainOutDataTypeStr=single  IProdOutDataTypeStr=single  IOutMin=[]  IOutMax=[]  DGainOutDataTypeStr=single  DProdOutDataTypeStr=single  DOutMin=[]  DOutMax=[]  NGainOutDataTypeStr=single  NProdOutDataTypeStr=single  NOutMin=[]  NOutMax=[]  SumOutDataTypeStr=single  SumOutMin=[]  SumOutMax=[]  SaturationOutMin=[]  SaturationOutMax=[]  PParamMin=[]  PParamMax=[]  IParamMin=[]  IParamMax=[]  DParamMin=[]  DParamMax=[]  NParamMin=[]  NParamMax=[]  KbParamMin=[]  KbParamMax=[]  KtParamMin=[]  KtParamMax=[]  KbOutMin=[]  KbOutMax=[]  KtOutMin=[]  KtOutMax=[]  IntegratorOutMin=[]  IntegratorOutMax=[]  FilterOutMin=[]  FilterOutMax=[]  SumI1OutMin=[]  SumI1OutMax=[]  SumI2OutMin=[]  SumI2OutMax=[]  SumI3OutMin=[]  SumI3OutMax=[]  SumI4OutMin=[]  SumI4OutMax=[]  SumDOutMin=[]  SumDOutMax=[]  DifferentiatorOutMin=[]  DifferentiatorOutMax=[]  FilterDiffOutCoefMin=[]  FilterDiffOutCoefMax=[]  ReciprocalOutMin=[]  ReciprocalOutMax=[]  SumDenOutMin=[]  SumDenOutMax=[]  SumNumOutMin=[]  SumNumOutMax=[]  DivideOutMin=[]  DivideOutMax=[]  UdiffTsProdOutMin=[]  UdiffTsProdOutMax=[]  NTsProdOutMin=[]  NTsProdOutMax=[]  UintegralTsProdOutMin=[]  UintegralTsProdOutMax=[]  UngainTsProdOutMin=[]  UngainTsProdOutMax=[]  ClampingZeroOutDataTypeStr=Inherit: Inherit via back propagation  ClampingZeroOutMin=[]  ClampingZeroOutMax=[]  FilterDenConstantOutDataTypeStr=Inherit: Inherit via back propagation  FilterDenConstantOutMin=[]  FilterDenConstantOutMax=[]  PCopyOutDataTypeStr=Inherit: Inherit via back propagation  PCopyOutMin=[]  PCopyOutMax=[]  NCopyOutDataTypeStr=Inherit: Inherit via back propagation  NCopyOutMin=[]  NCopyOutMax=[]  IntegratorContinuousStateAttributes=''  IntegratorStateMustResolveToSignalObject=off  IntegratorRTWStateStorageClass=Auto  FilterContinuousStateAttributes=''  FilterStateMustResolveToSignalObject=off  FilterRTWStateStorageClass=Auto  ParallelPVariant=InternalParameters  IdealPVariant=Disabled  IVariant=InternalParameters  DVariant=InternalParameters  IntegratorVariant=Discrete  SatVariant=Enabled  AWVariant=DiscClampingParallel  PCopyVariant=Disabled  TRVariant=Disabled  FdbkBlocksVariant=Forward  IdealPFdbkVariant=Disabled  SatFdbkVariant=Disabled  DerivativeFilterVariant=ForwardEulerFilter  NVariant=InternalParameters  NCopyVariant=Disabled  FilterICVariant=InternalICsFilter  IntegratorICVariant=InternalICs  ExternalResetVariant=Disabled  TRSumVariant=Passthrough  SumFdbkVariant=Disabled  SumVariant=Sum_PID  TsampFilterVariant=InternalTs  TsampNgainVariant=Passthrough  TsampIntegralVariant=Disabled_SignalSpec  ExternalSaturationOutDataTypeStr=Inherit: Same as second input  DerivativeSourceVariant=ErrorSignal
  Sum : Sum  Inputs=|+-
  Sum1 : Sum  Inputs=|+-
  Sum4 : Sum  Inputs=|+-
  tau_roll : Outport
  tau_pitch : Outport  Port=2
  tau_yaw : Outport  Port=3
  log_att : Outport  Port=4
  wires:
  PID Controller6/1 -> tau_yaw/1
  [des_r] -> Gain4/1
  Gain4/1 -> Mux/5
  Gain3/1 -> Mux/4
  Gain6/1 -> Mux/7
  [des_q] -> Gain3/1
  [pqr] -> Gain6/1
  PID Controller2/1 -> tau_roll/1
  [des_p] -> Gain2/1
  Gain2/1 -> Mux/3
  Mux/1 -> log_att/1
  Gain15/1 -> Mux/1
  PID Controller1/1 -> tau_pitch/1
  Gain1/1 -> Mux/2
  des_r/1 -> [des_r], Sum4/1
  Sum4/1 -> PID Controller6/1
  Demux/3 -> Sum4/2
  Sum/1 -> PID Controller1/1
  [RPY] -> Gain5/1
  Demux/2 -> Sum/2
  [des_R] -> Gain15/1
  [des_P] -> Gain1/1
  Demux/1 -> Sum1/2
  pqr/1 -> [pqr], Demux/1
  Sum1/1 -> PID Controller2/1
  Gain5/1 -> Mux/6
  des_p/1 -> [des_p], Sum1/1
  des_q/1 -> [des_q], Sum/1

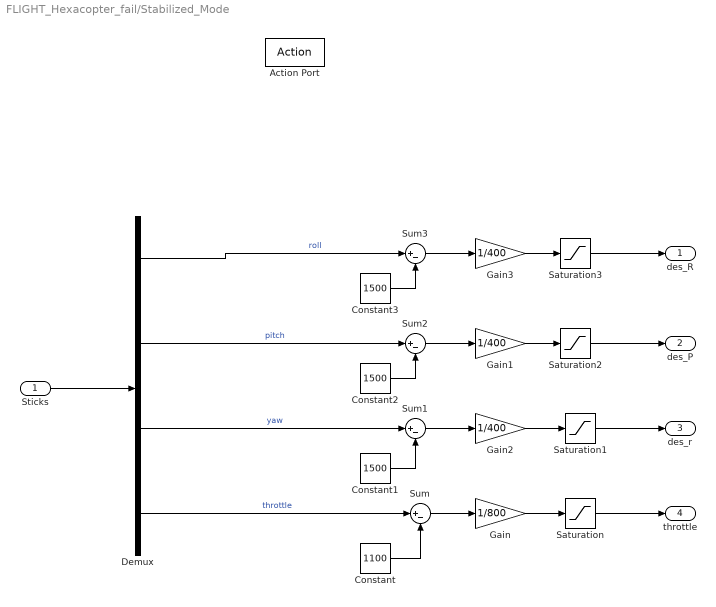
== system FLIGHT_Hexacopter_fail/Stabilized_Mode ==
  Sticks : Inport
  Action Port : ActionPort  ActionPortLabel=else
  Constant : Constant  Value=1100
  Constant1 : Constant  Value=1500  OutDataTypeStr=single
  Constant2 : Constant  Value=1500  OutDataTypeStr=single
  Constant3 : Constant  Value=1500  OutDataTypeStr=single
  Demux : Demux
  Gain : Gain  Gain=1/800  OutDataTypeStr=single
  Gain1 : Gain  Gain=1/400  OutDataTypeStr=single
  Gain2 : Gain  Gain=1/400  OutDataTypeStr=single
  Gain3 : Gain  Gain=1/400  OutDataTypeStr=single
  Saturation : Saturate  UpperLimit=0.90  LowerLimit=0
  Saturation1 : Saturate  UpperLimit=1  LowerLimit=-1
  Saturation2 : Saturate  UpperLimit=1  LowerLimit=-1
  Saturation3 : Saturate  UpperLimit=1  LowerLimit=-1
  Sum{,1..3} (4 alike) : Sum  Inputs=|+-
  des_R : Outport
  des_P : Outport  Port=2
  des_r : Outport  Port=3
  throttle : Outport  Port=4
  wires:
  Demux/1 -> Sum3/1  "roll"
  Gain3/1 -> Saturation3/1
  Constant1/1 -> Sum1/2
  Gain/1 -> Saturation/1
  Demux/2 -> Sum2/1  "pitch"
  Gain2/1 -> Saturation1/1
  Demux/4 -> Sum/1  "throttle"
  Constant3/1 -> Sum3/2
  Sum3/1 -> Gain3/1
  Constant/1 -> Sum/2
  Saturation2/1 -> des_P/1
  Sum1/1 -> Gain2/1
  Gain1/1 -> Saturation2/1
  Constant2/1 -> Sum2/2
  Saturation3/1 -> des_R/1
  Saturation/1 -> throttle/1
  Demux/3 -> Sum1/1  "yaw"
  Sum/1 -> Gain/1
  Sum2/1 -> Gain1/1
  Saturation1/1 -> des_r/1
  Sticks/1 -> Demux/1

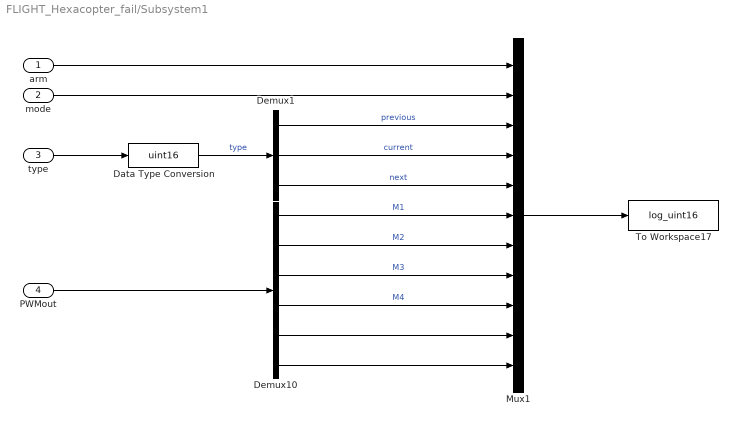
== system FLIGHT_Hexacopter_fail/Subsystem1 ==
  arm : Inport
  mode : Inport  Port=2
  type : Inport  Port=3
  PWMout : Inport  Port=4
  Data Type Conversion : DataTypeConversion  OutDataTypeStr=uint16  SaturateOnIntegerOverflow=off  RndMeth=Floor
  Demux1 : Demux  Outputs=3
  Demux10 : Demux  Outputs=6
  Mux1 : Mux  Inputs=11
  To Workspace17 : ToWorkspace  VariableName=log_uint16  SaveFormat=Structure With Time  SampleTime=SampleTime
      settings: Save2DSignal=2-D array (concatenate along first dimension)
  wires:
  Mux1/1 -> To Workspace17/1
  PWMout/1 -> Demux10/1
  type/1 -> Data Type Conversion/1
  arm/1 -> Mux1/1
  mode/1 -> Mux1/2
  Demux1/3 -> Mux1/5  "next"
  Demux1/2 -> Mux1/4  "current"
  Demux1/1 -> Mux1/3  "previous"
  Data Type Conversion/1 -> Demux1/1  "type"
  Demux10/1 -> Mux1/6  "M1"
  Demux10/2 -> Mux1/7  "M2"
  Demux10/3 -> Mux1/8  "M3"
  Demux10/4 -> Mux1/9  "M4"
  Demux10/5 -> Mux1/10
  Demux10/6 -> Mux1/11

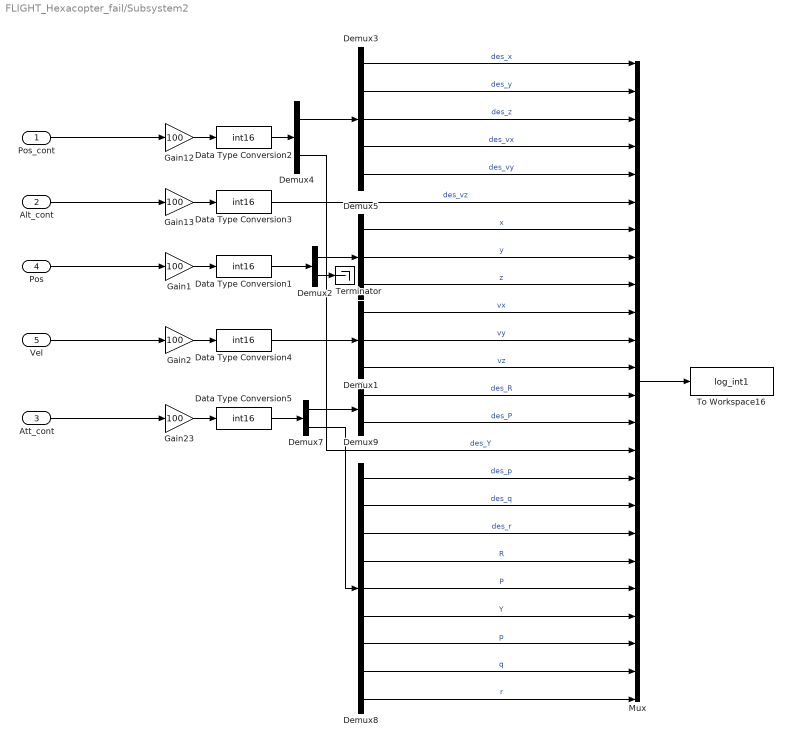
== system FLIGHT_Hexacopter_fail/Subsystem2 ==
  Pos_cont : Inport
  Alt_cont : Inport  Port=2
  Att_cont : Inport  Port=3
  Pos : Inport  Port=4
  Vel : Inport  Port=5
  Data Type Conversion{1..5} (5 alike) : DataTypeConversion  OutDataTypeStr=int16  SaturateOnIntegerOverflow=off  RndMeth=Floor
  Demux1 : Demux  Outputs=3
  Demux2 : Demux  Outputs=[3 1]
  Demux3 : Demux  Outputs=5
  Demux4 : Demux  Outputs=[5 1]
  Demux5 : Demux  Outputs=3
  Demux7 : Demux  Outputs=[2 9]
  Demux8 : Demux  Outputs=9
  Demux9 : Demux  Outputs=2
  Gain{1..2,12..13,23} (5 alike) : Gain  Gain=100
  Mux : Mux  Inputs=24
  Terminator : Terminator
  To Workspace16 : ToWorkspace  VariableName=log_int1  SaveFormat=Structure  SampleTime=SampleTime
      settings: Save2DSignal=2-D array (concatenate along first dimension)
  wires:
  Att_cont/1 -> Gain23/1
  Data Type Conversion5/1 -> Demux7/1
  Data Type Conversion3/1 -> Mux/6  "des_vz"
  Data Type Conversion2/1 -> Demux4/1
  Demux2/2 -> Terminator/1
  Demux2/1 -> Demux5/1
  Data Type Conversion1/1 -> Demux2/1
  Data Type Conversion4/1 -> Demux1/1
  Gain2/1 -> Data Type Conversion4/1
  Demux1/3 -> Mux/12  "vz"
  Demux1/2 -> Mux/11  "vy"
  Demux1/1 -> Mux/10  "vx"
  Vel/1 -> Gain2/1
  Gain1/1 -> Data Type Conversion1/1
  Pos/1 -> Gain1/1
  Demux8/8 -> Mux/23  "q"
  Demux8/2 -> Mux/17  "des_q"
  Demux3/5 -> Mux/5  "des_vy"
  Demux8/9 -> Mux/24  "r"
  Gain23/1 -> Data Type Conversion5/1
  Demux5/3 -> Mux/9  "z"
  Demux5/2 -> Mux/8  "y"
  Mux/1 -> To Workspace16/1
  Demux3/1 -> Mux/1  "des_x"
  Pos_cont/1 -> Gain12/1
  Demux8/7 -> Mux/22  "p"
  Demux3/3 -> Mux/3  "des_z"
  Demux8/6 -> Mux/21  "Y"
  Demux4/1 -> Demux3/1
  Demux7/2 -> Demux8/1
  Demux7/1 -> Demux9/1
  Demux9/1 -> Mux/13  "des_R"
  Demux3/4 -> Mux/4  "des_vx"
  Alt_cont/1 -> Gain13/1
  Demux4/2 -> Mux/15  "des_Y"
  Demux8/3 -> Mux/18  "des_r"
  Demux3/2 -> Mux/2  "des_y"
  Demux8/1 -> Mux/16  "des_p"
  Gain12/1 -> Data Type Conversion2/1
  Demux8/5 -> Mux/20  "P"
  Demux5/1 -> Mux/7  "x"
  Demux8/4 -> Mux/19  "R"
  Gain13/1 -> Data Type Conversion3/1
  Demux9/2 -> Mux/14  "des_P"

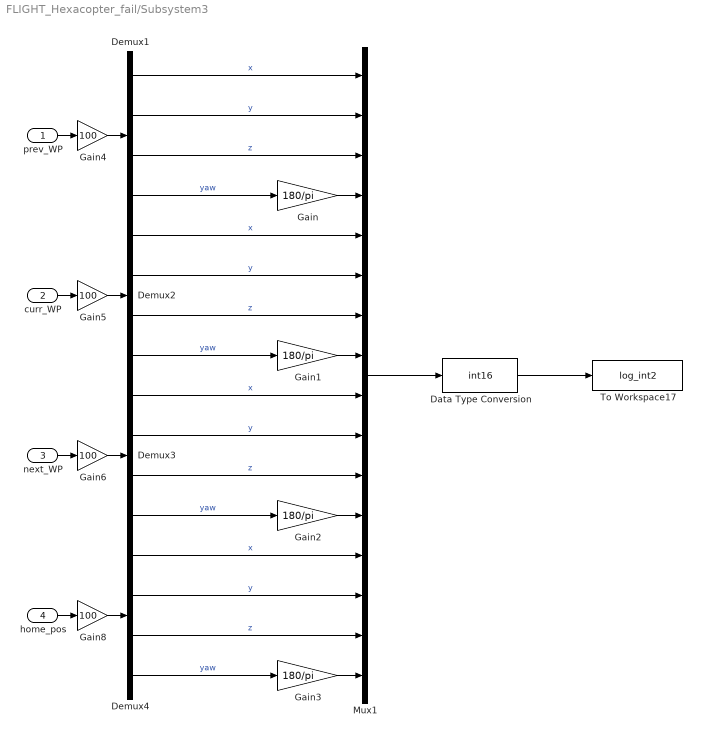
== system FLIGHT_Hexacopter_fail/Subsystem3 ==
  prev_WP : Inport
  curr_WP : Inport  Port=2
  next_WP : Inport  Port=3
  home_pos : Inport  Port=4
  Data Type Conversion : DataTypeConversion  OutDataTypeStr=int16  SaturateOnIntegerOverflow=off  RndMeth=Floor
  Demux{1..4} (4 alike) : Demux
  Gain{,1..3} (4 alike) : Gain  Gain=180/pi
  Gain{4..6,8} (4 alike) : Gain  Gain=100
  Mux1 : Mux  Inputs=16
  To Workspace17 : ToWorkspace  VariableName=log_int2  SaveFormat=Structure  SampleTime=SampleTime
      settings: Save2DSignal=2-D array (concatenate along first dimension)
  wires:
  Mux1/1 -> Data Type Conversion/1
  Demux1/4 -> Gain/1  "yaw"
  prev_WP/1 -> Gain4/1
  Demux1/1 -> Mux1/1  "x"
  Demux1/2 -> Mux1/2  "y"
  Demux1/3 -> Mux1/3  "z"
  Demux2/4 -> Gain1/1  "yaw"
  Demux2/3 -> Mux1/7  "z"
  Demux2/1 -> Mux1/5  "x"
  Demux2/2 -> Mux1/6  "y"
  Demux3/4 -> Gain2/1  "yaw"
  Demux3/3 -> Mux1/11  "z"
  Demux3/1 -> Mux1/9  "x"
  Demux3/2 -> Mux1/10  "y"
  Demux4/4 -> Gain3/1  "yaw"
  Demux4/3 -> Mux1/15  "z"
  Demux4/1 -> Mux1/13  "x"
  Demux4/2 -> Mux1/14  "y"
  curr_WP/1 -> Gain5/1
  next_WP/1 -> Gain6/1
  home_pos/1 -> Gain8/1
  Gain4/1 -> Demux1/1
  Gain5/1 -> Demux2/1
  Gain6/1 -> Demux3/1
  Gain8/1 -> Demux4/1
  Gain/1 -> Mux1/4
  Gain1/1 -> Mux1/8
  Gain2/1 -> Mux1/12
  Gain3/1 -> Mux1/16
  Data Type Conversion/1 -> To Workspace17/1

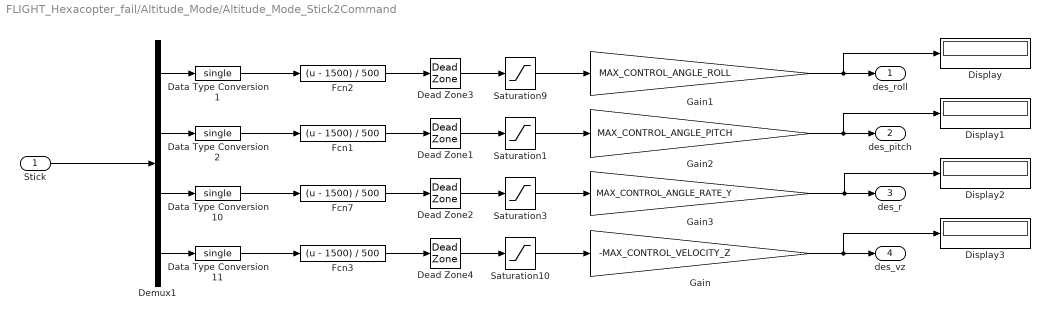
== system FLIGHT_Hexacopter_fail/Altitude_Mode/Altitude_Mode_Stick2Command ==
  Stick : Inport
  Data Type Conversion{1..2,10..11} (4 alike) : DataTypeConversion  OutDataTypeStr=single  SaturateOnIntegerOverflow=off  RndMeth=Floor
  Dead Zone1 : DeadZone  LowerValue=-0.001  UpperValue=0.001
  Dead Zone2 : DeadZone  LowerValue=-0.005  UpperValue=0.005
  Dead Zone3 : DeadZone  LowerValue=-0.003  UpperValue=0.003
  Dead Zone4 : DeadZone  LowerValue=-0.03  UpperValue=0.03
  Demux1 : Demux
  Display{,1..3} (4 alike) : Display
  Fcn{1..3,7} (4 alike) : Fcn  Expr=(u - 1500) / 500
  Gain : Gain  Gain=-MAX_CONTROL_VELOCITY_Z
  Gain1 : Gain  Gain=MAX_CONTROL_ANGLE_ROLL
  Gain2 : Gain  Gain=MAX_CONTROL_ANGLE_PITCH
  Gain3 : Gain  Gain=MAX_CONTROL_ANGLE_RATE_Y
  Saturation{1,3,9..10} (4 alike) : Saturate  UpperLimit=1  LowerLimit=-1
  des_roll : Outport
  des_pitch : Outport  Port=2
  des_r : Outport  Port=3
  des_vz : Outport  Port=4
  wires:
  Fcn3/1 -> Dead Zone4/1
  Saturation10/1 -> Gain/1
  Gain1/1 -> Display/1, des_roll/1
  Fcn1/1 -> Dead Zone1/1
  Data Type Conversion1/1 -> Fcn2/1
  Gain2/1 -> Display1/1, des_pitch/1
  Saturation1/1 -> Gain2/1
  Data Type Conversion11/1 -> Fcn3/1
  Dead Zone4/1 -> Saturation10/1
  Gain3/1 -> Display2/1, des_r/1
  Demux1/1 -> Data Type Conversion1/1
  Dead Zone1/1 -> Saturation1/1
  Saturation9/1 -> Gain1/1
  Saturation3/1 -> Gain3/1
  Demux1/4 -> Data Type Conversion11/1
  Data Type Conversion10/1 -> Fcn7/1
  Fcn2/1 -> Dead Zone3/1
  Stick/1 -> Demux1/1
  Demux1/2 -> Data Type Conversion2/1
  Dead Zone3/1 -> Saturation9/1
  Dead Zone2/1 -> Saturation3/1
  Fcn7/1 -> Dead Zone2/1
  Data Type Conversion2/1 -> Fcn1/1
  Demux1/3 -> Data Type Conversion10/1
  Gain/1 -> Display3/1, des_vz/1

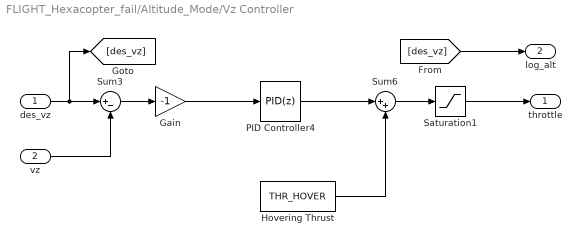
== system FLIGHT_Hexacopter_fail/Altitude_Mode/Vz Controller ==
  des_vz : Inport
  vz : Inport  Port=2
  Gain : Gain  Gain=-1
  Hovering Thrust : Constant  Value=THR_HOVER  OutDataTypeStr=single  SampleTime=SampleTime
  PID Controller4 : slpidlib/PID Controller  Controller=PID  Form=Parallel  TimeDomain=Discrete-time  UseExternalTs=off  SampleTime=SampleTime  IntegratorMethod=Forward Euler  FilterMethod=Forward Euler  ControllerParametersSource=internal  P=Kpvz  I=Kivz  UseKiTs=off  D=Kdvz  UseExternalDerivativeSource=off  N=Nvz  UseFilter=on  TunerSelectOption=Transfer Function Based (PID Tuner App)  InitialConditionSource=internal  InitialConditionForIntegrator=0  InitialConditionForFilter=0  DifferentiatorICPrevScaledInput=0  ExternalReset=none  TrackingMode=off  Kt=1  LimitOutput=on  SatLimitsSource=internal  UpperSaturationLimit=1  LowerSaturationLimit=-1  LinearizeAsGain=on  AntiWindupMode=clamping  Kb=1  LimitIntegrator=off  UpperIntegratorSaturationLimit=inf  LowerIntegratorSaturationLimit=-inf  POutMin=[]  POutMax=[]  IOutMin=[]  IOutMax=[]  DOutMin=[]  DOutMax=[]  NOutMin=[]  NOutMax=[]  SumOutMin=[]  SumOutMax=[]  SaturationOutMin=[]  SaturationOutMax=[]  PParamMin=[]  PParamMax=[]  IParamMin=[]  IParamMax=[]  DParamMin=[]  DParamMax=[]  NParamMin=[]  NParamMax=[]  KbParamMin=[]  KbParamMax=[]  KtParamMin=[]  KtParamMax=[]  KbOutMin=[]  KbOutMax=[]  KtOutMin=[]  KtOutMax=[]  IntegratorOutMin=[]  IntegratorOutMax=[]  FilterOutMin=[]  FilterOutMax=[]  SumI1OutMin=[]  SumI1OutMax=[]  SumI2OutMin=[]  SumI2OutMax=[]  SumI3OutMin=[]  SumI3OutMax=[]  SumI4OutMin=[]  SumI4OutMax=[]  SumDOutMin=[]  SumDOutMax=[]  DifferentiatorOutMin=[]  DifferentiatorOutMax=[]  FilterDiffOutCoefMin=[]  FilterDiffOutCoefMax=[]  ReciprocalOutMin=[]  ReciprocalOutMax=[]  SumDenOutMin=[]  SumDenOutMax=[]  SumNumOutMin=[]  SumNumOutMax=[]  DivideOutMin=[]  DivideOutMax=[]  UdiffTsProdOutMin=[]  UdiffTsProdOutMax=[]  NTsProdOutMin=[]  NTsProdOutMax=[]  UintegralTsProdOutMin=[]  UintegralTsProdOutMax=[]  UngainTsProdOutMin=[]  UngainTsProdOutMax=[]  ClampingZeroOutDataTypeStr=Inherit: Inherit via back propagation  ClampingZeroOutMin=[]  ClampingZeroOutMax=[]  FilterDenConstantOutDataTypeStr=Inherit: Inherit via back propagation  FilterDenConstantOutMin=[]  FilterDenConstantOutMax=[]  PCopyOutDataTypeStr=Inherit: Inherit via back propagation  PCopyOutMin=[]  PCopyOutMax=[]  NCopyOutDataTypeStr=Inherit: Inherit via back propagation  NCopyOutMin=[]  NCopyOutMax=[]  IntegratorContinuousStateAttributes=''  IntegratorStateMustResolveToSignalObject=off  IntegratorRTWStateStorageClass=Auto  FilterContinuousStateAttributes=''  FilterStateMustResolveToSignalObject=off  FilterRTWStateStorageClass=Auto  ParallelPVariant=InternalParameters  IdealPVariant=Disabled  IVariant=InternalParameters  DVariant=InternalParameters  IntegratorVariant=Discrete  SatVariant=Enabled  AWVariant=DiscClampingParallel  PCopyVariant=Disabled  TRVariant=Disabled  FdbkBlocksVariant=Forward  IdealPFdbkVariant=Disabled  SatFdbkVariant=Disabled  DerivativeFilterVariant=ForwardEulerFilter  NVariant=InternalParameters  NCopyVariant=Disabled  FilterICVariant=InternalICsFilter  IntegratorICVariant=InternalICs  ExternalResetVariant=Disabled  TRSumVariant=Passthrough  SumFdbkVariant=Disabled  SumVariant=Sum_PID  TsampFilterVariant=InternalTs  TsampNgainVariant=Passthrough  TsampIntegralVariant=Disabled_SignalSpec  ExternalSaturationOutDataTypeStr=Inherit: Same as second input  DerivativeSourceVariant=ErrorSignal
  Saturation1 : Saturate  UpperLimit=1  LowerLimit=0  OutDataTypeStr=single
  Sum3 : Sum  Inputs=|+-
  Sum6 : Sum  Inputs=|++  OutDataTypeStr=single
  throttle : Outport  OutDataTypeStr=single
  log_alt : Outport  Port=2  OutDataTypeStr=single
  wires:
  Saturation1/1 -> throttle/1
  vz/1 -> Sum3/2
  des_vz/1 -> [des_vz], Sum3/1
  Sum3/1 -> Gain/1
  Gain/1 -> PID Controller4/1
  PID Controller4/1 -> Sum6/1
  Sum6/1 -> Saturation1/1
  Hovering Thrust/1 -> Sum6/2
  [des_vz] -> log_alt/1

== matlab function FLIGHT_Hexacopter_fail/quat2eul ==
  data: q input; ypr output
function ypr  = quat2eul(q)

% Quaternion conversion to Euler angles based on the PX4 Firmware v1.10.2
% release.

phi = atan2(2*(q(1)*q(2) + q(3)* q(4)), q(1)^2 - q(2)^2 - q(3)^2 + q(4)^2);
theta = asin(-2*(q(2)*q(4) - q(1)*q(3)));
psi = atan2(2*(q(2)*q(3) + q(1)* q(4)), q(1)^2 + q(2)^2 - q(3)^2 - q(4)^2);

ypr = [psi theta phi];

end
